simulink model "consolidated_sensors_deploy"  (R2025b)
settings: Solver=FixedStepAuto  StartTime=0.0  StopTime=10.0  RelTol=1e-3  EnableMultiTasking=on
settings Model: ExtModeTrigDuration=2  Creator=atcushen  LastModifiedBy=atcushen
settings SolverCC: PositivePriorityOrder=on
settings OptimizationCC: EnhancedBackFolding=on  PassReuseOutputArgsAs=Individual arguments  ZeroExternalMemoryAtStartup=off  ZeroInternalMemoryAtStartup=off  MaxStackSize=200000  OptimizeBlockOrder=speed  DifferentSizesBufferReuse=on  OptimizationCustomize=off  EfficientTunableParamExpr=on
settings DebuggingCC: ParameterTunabilityLossMsg=error
settings HardwareCC: ProdBitPerPointer=32.0  ProdBitPerSizeT=32.0  ProdBitPerPtrDiffT=32.0  ProdLargestAtomicInteger=Long  ProdLargestAtomicFloat=Double  ProdWordSize=32.0  ProdLongLongMode=on  ProdHWDeviceType=ARM Compatible->ARM Cortex-A (32-bit)  UseEmbeddedCoderFeatures=off  UseSimulinkCoderFeatures=off
settings RTWCC: SystemTargetFile=ert.tlc  HardwareBoard=Raspberry Pi  TLCOptions="-aInlineSetEventsForThisBaseRateFcn=TLC_FALSE -aSuppressMultiTaskScheduler=TLC_FALSE  -aRateBasedStepFcn=0"  TemplateMakefile=ert_default_tmf  Toolchain=GNU GCC Embedded Linux  BuildConfiguration=Faster Runs  Description=Embedded Coder
settings CodeAppCC: ForceParamTrailComments=on  IgnoreCustomStorageClasses=off  OperatorAnnotations=on  SimulinkDataObjDesc=on  SFDataObjDesc=on  InsertBlockDesc=on
settings ERTTargetCC: ExtModeTransport=2.0  ExtModeStaticAlloc=on  ExtModeMexFile=ext_xcp  ExtModeIntrfLevel=Level2 - Open  InlinedParameterPlacement=Hierarchical  SupportNonInlinedSFcns=on  SupportVariableSizeSignals=on

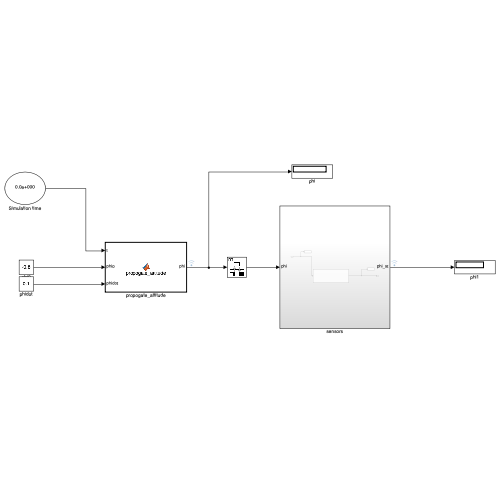
[thumbnail: Simulink's stored preview of the top-level diagram]
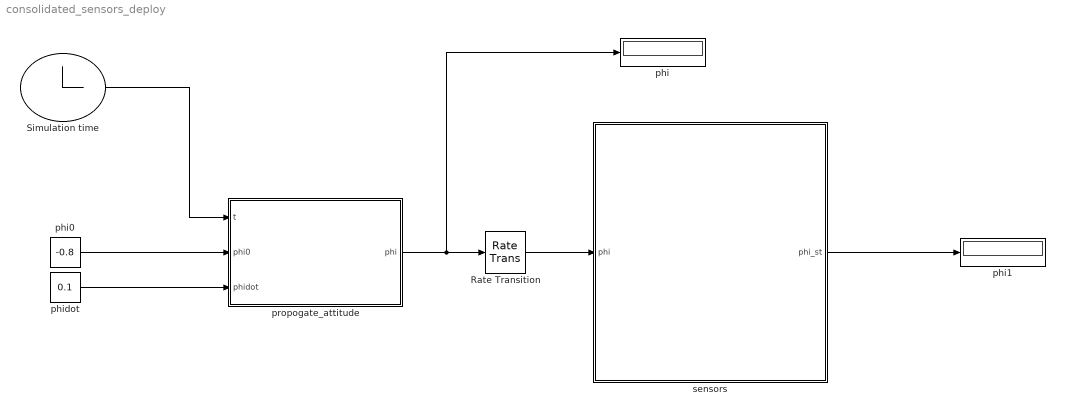
== system consolidated_sensors_deploy ==
  Rate Transition : RateTransition  OutPortSampleTime=0.1
  Simulation time : Clock
  phi : Display
  phi0 : Constant  Value=-0.8
  phi1 : Display
  phidot : Constant  Value=0.1
  propogate_attitude : MATLAB Function  TreatAsAtomicUnit=on
  sensors : Subsystem
  wires:
  Simulation time/1 -> propogate_attitude/1(t)
  propogate_attitude/1(phi) -> phi/1, Rate Transition/1
  phi0/1 -> propogate_attitude/2(phi0)
  phidot/1 -> propogate_attitude/3(phidot)
  Rate Transition/1 -> sensors/1(phi)
  sensors/1(phi_st) -> phi1/1

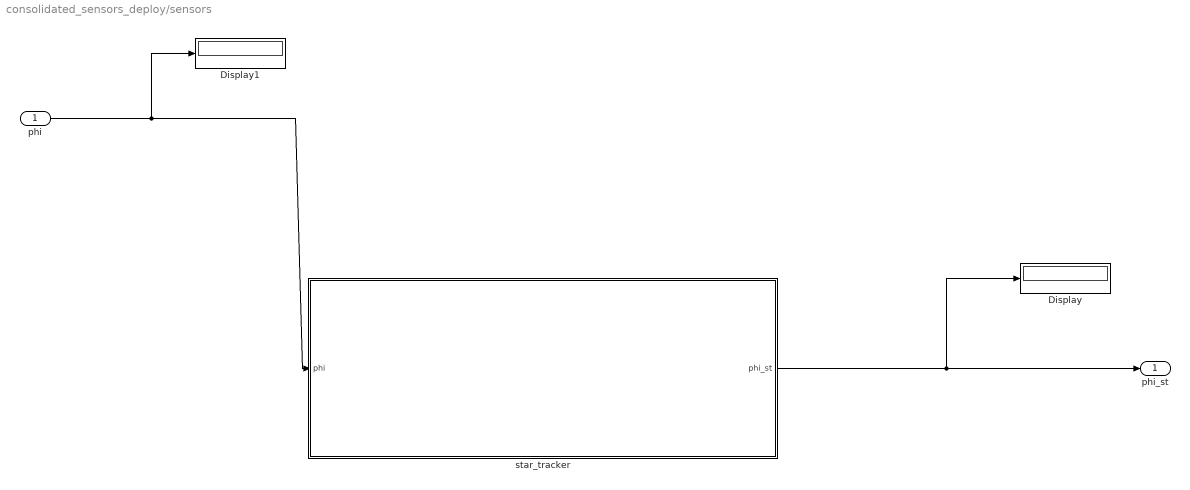
== system consolidated_sensors_deploy/sensors ==
  phi : Inport
  Display : Display
  Display1 : Display
  star_tracker : Subsystem
  phi_st : Outport
  wires:
  phi/1 -> Display1/1, star_tracker/1(phi)
  star_tracker/1(phi_st) -> Display/1, phi_st/1

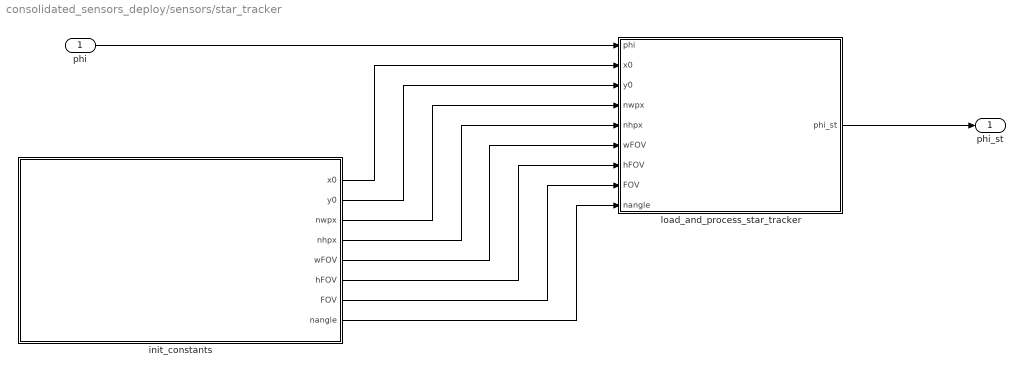
== system consolidated_sensors_deploy/sensors/star_tracker ==
  phi : Inport
  init_constants : MATLAB Function  TreatAsAtomicUnit=on
  load_and_process_star_tracker : MATLAB Function  TreatAsAtomicUnit=on
  phi_st : Outport
  wires:
  load_and_process_star_tracker/1(phi_st) -> phi_st/1
  init_constants/1(x0) -> load_and_process_star_tracker/2(x0)
  phi/1 -> load_and_process_star_tracker/1(phi)
  init_constants/2(y0) -> load_and_process_star_tracker/3(y0)
  init_constants/3(nwpx) -> load_and_process_star_tracker/4(nwpx)
  init_constants/4(nhpx) -> load_and_process_star_tracker/5(nhpx)
  init_constants/5(wFOV) -> load_and_process_star_tracker/6(wFOV)
  init_constants/6(hFOV) -> load_and_process_star_tracker/7(hFOV)
  init_constants/7(FOV) -> load_and_process_star_tracker/8(FOV)
  init_constants/8(nangle) -> load_and_process_star_tracker/9(nangle)

== matlab function consolidated_sensors_deploy/propogate_attitude ==
  data: t input; phi output; phi0 input; phidot input
% propogate attitude
function phi = propogate_attitude(t,phi0,phidot)
    % Input: 
    % t: float, current time, in s
    % phi0: float, initial attitude, in radians
    % phidot: float, rotation rate, in rad/sec
    
    % Output:
    % phi: float, current attitude, in rad/sec

    phi = mod(t*phidot + phi0 + pi,2*pi) - pi;
    %disp(['Propogated attitude at t = ',num2str(t),' to phi = ',num2str(phi)]);
end

== matlab function consolidated_sensors_deploy/sensors/star_tracker/load_and_process_star_tracker ==
  data: phi_st output; phi input; x0 input; y0 input; nwpx input; nhpx input; wFOV input; hFOV input; FOV input; nangle input
function phi_st  = load_and_process_star_tracker(phi,x0,y0,nwpx,nhpx,wFOV,hFOV,FOV,nangle)
    
    % DEFINE PATHS TO STARFIELD IMAGE AND STARTABLE
    starfield_path = 'star_field.mat'; % str, name of reference photo of full starfield image (which nwpx,wFOV etc describe)
    startable_path = 'star_table.mat'; % str, name of table which identifies star locations, in radians 


    % PART 1: IMPORT STAR TABLE

    struct = coder.load(startable_path);
    star_table = struct.star_table;
    

    
    % PART 2: GENERATE LOOKUP TABLE

    % Initialize lookup table
    star_lookup = zeros(size(star_table, 1), nangle);

    % Iterate through each star in the table
    for istar = 1:length(star_table)
        
        % Compute the angular distances from the current star to all other stars
        phi_diff = star_table(istar, 1) - star_table(:, 1);
        theta_diff = star_table(istar, 2) - star_table(:, 2);
        angle_diff = sqrt(phi_diff.^2 + theta_diff.^2);

        % Sort the angular distances and get the indices of the smallest values
        [sorted_angles, ~] = sort(angle_diff);
        star_lookup(istar, :) = sorted_angles(2:min(nangle+1, length(sorted_angles))); % Store the smallest values
    end

    
    % PART 3: LOAD AND CROP IMAGE

    % Input
    % image: str, path to .png field to import of starfield
    % phi: float, boresight angle of camera, in radians, from -pi to pis
    % FOV: float, angular field of view of camera, in radians, from 0 to 2pi
    % x0: int, x pixel coord of reference star 
    % y0: int, x pixel coord of reference star 
    % nwpx: int, number of pixels of width of starfield image
    % nhpx: int, number of pixels of height of starfield image
    % wFOV: float, field of view width of starfield image [deg]
    % hFOV: float, field of view height of starfield image [deg]
    % Output:
    % st_im: nres x nres array, representing synethic star tracker image

    % Load the .png image as a black and white image array
    file = coder.load(starfield_path);
    img = file.img; 
    starfield_im = rgb2gray(img); % Convert the image to grayscale
    starfield_im = flip(starfield_im,1); % Image array is upside down)

    % Create coordinate axes
    x_ax = linspace(1,nwpx,nwpx) - x0;
    y_ax = linspace(1,nhpx,nhpx) - y0;
    phi_ax = x_ax * pi/180 * wFOV/nwpx;
    theta_ax = y_ax * pi/180 * hFOV/nhpx;
    
    % Crop the starfield image based on the field of view and the phi axis
    phi_indices = phi_ax >= (phi - FOV/2) & phi_ax <= (phi + FOV/2);
    theta_indices = theta_ax >= (-FOV/2) & theta_ax <= (FOV/2); %y0-round(nres/2):y0-round(nres/2)+nres-1;
    
    % Ensure indices are within bounds
    %phi_indices = max(min(phi_indices, nwpx), 1);
    %theta_indices = max(min(theta_indices, nhpx), 1);
    
    % Crop the image
    st_im = starfield_im(theta_indices, phi_indices);

    
    % PART 4: LOCATE STARS

    % Input:
    % st_im: nxn array, representing image from star tracker
    % FOV: float, field of view along each edge of image
    % Output:
    % star_ls: nx2 array, the phi and theta positions (relative to the
    % center of the image) for each star identified
    
    % Get image dimensions (not passed to function call)
    [theta_nres,phi_nres] = size(st_im);
    
    % Convert coordinates to phi and theta positions
    phi_positions = linspace(-FOV/2, FOV/2, phi_nres);
    theta_positions = linspace(-FOV/2, FOV/2, theta_nres);
    
    % Identify bright points in the star tracker image
     threshold = 0.3 * 255; % Set a threshold to identify bright points
    % Create filtered im
     filtered_im = zeros(size(st_im)); % Initialize filtered image
     filtered_im(st_im > threshold) = 1; % Set values to 1 where st_im exceeds threshold
    % Find connected components
     CC = bwconncomp(filtered_im);
    % Create label matrix - CHANGED FOR CODEGEN
     L = zeros(size(filtered_im), 'uint16');
     for k = 1:CC.NumObjects
         L(CC.PixelIdxList{k}) = k;
     end
    % Create output array for star positions
     star_ls = zeros(max(L(:)), 2);
    % Iterate through each connected component
    for istar = 1:max(L(:))
    % Get the coordinates of the current star cluster
     [y_cluster, x_cluster] = find(L == istar);
    % Store the average position of the cluster
     star_ls(istar, 1) = mean(phi_positions(x_cluster)); % Average phi coordinate
     star_ls(istar, 2) = mean(theta_positions(y_cluster)); % Average theta coordinate
    end
    

    % PART 5: MATCH STARS TO LOOKUP TABLE

    star_pos_error = 10*wFOV/nwpx*pi/180;

    % Input
    % star_ls: nx2 array, the phi and theta positions (relative to the
    % center of the image) for each star identified
    % star_pos_error: float, angular uncertainty in position of stars
    % star_lookup: nxnagle array, each row corresponds to given row in
    % star_table, columns are angular distances to closest stars

    % Output
    % star_num: integer, index number of matched star
    % deltaphi: float, offset in phi of matched star from image center, in
    % radians
    % deltatheta: float, offset in phi of matched star from image center,
    % in radians
    % CHANGED FOR CODEGEN - Initialize outputs with default values
    star_num = int32(-1);
    deltaphi = 0.0;
    deltatheta = 0.0;
    match_status = int32(0);  % debug output
    stars_tried = int32(0);   % debug output

    % Iterate through stars in image, starting closest to middle, until we
    % get a positive match
    star_match = false;
    
    % Calculate the sum of squares for each star position
    star_ls_dist = sum(star_ls.^2, 2);
    
    % Sort the star_ls based on the sum of squares
    [~, sorted_indices] = sort(star_ls_dist);
    star_ls = star_ls(sorted_indices, :);

    istar = 1;
    while star_match == false && istar <= length(star_ls)
        stars_tried = int32(istar);  % tracking progress
        
        % Compute distances to other stars
        phi_diff = star_ls(istar, 1) - star_ls(:, 1);
        theta_diff = star_ls(istar, 2) - star_ls(:, 2);
        angle_diff = sqrt(phi_diff.^2 + theta_diff.^2);

        % Sort the computed angular distances from smallest to largest
        [sorted_angles, ~] = sort(angle_diff);
        
        % Drop the first element of sorted_angles (distance to itself = 0)
        sorted_angles(1) = [];

        % Reduce sorted angles to only be as long as star_lookup is wide
        sorted_angles = sorted_angles(1:min(length(sorted_angles), size(star_lookup, 2)));

        % Create an array of stars within the positional error range
        match_indices = star_lookup(:, 1) >= (sorted_angles(1) - star_pos_error) & ...
                        star_lookup(:, 1) <= (sorted_angles(1) + star_pos_error);
        matched_stars = star_lookup(match_indices, :);

        % Check if that immediately identified the current state. 
        % If not, compare the angular distances one by one, bringing in more to
        % reduce the number of remaining options
        iangle = 2;

        while size(matched_stars,1) > 1 & iangle <= size(star_lookup,2)
            match_status = int32(2);  % indicates multiple matches being refined
            
            % We loop through the remaining matches
            for j = 1:size(match_indices, 1)
                if j ~= 0
                    % Check to see if the next closest star is within error of
                    % any of the neighbouring stars listed in the lookup table
                    % If none of the angles are close enough, then reject this
                    % match
                    if all(abs(star_lookup(j, iangle:end) - sorted_angles(iangle)) > star_pos_error)
                        match_indices(j) = 0; % Set the jth non-zero element of match_indices to zero
                    end
                end 
            end
            matched_stars = star_lookup(match_indices, :);
        
            iangle = iangle + 1;
        end
        
        % Check if we could use this star 
        if size(matched_stars,1) ~= 1
            % no match found for this star, continue
            istar = istar + 1; % Move to the next star
        else
            % CHANGED FOR CODEGEN - Force scalar by using loop instead of find
            for k = 1:length(match_indices)
                if match_indices(k) ~= 0
                    star_num = int32(k)
                    break;
                end
            end
            deltaphi = star_ls(istar,1); % Offset in phi
            deltatheta = star_ls(istar,2); % Offset in theta
            star_match = true;
            match_status = int32(1);  % successful match
        end
    end
    
    % Return error if star tracker failed 
    if star_match == false
        % CHANGED FOR CODEGEN - tracker failed
        star_num = int32(-1);
        deltaphi = 0.0;
        deltatheta = 0.0;
        match_status = int32(0);  % Failed to match
    end


    % FINALLY, COMPUTE PHI_ST

    if star_num<0
        phi_st = NaN;
    else
        phi_st = star_table(star_num,1) - deltaphi;
    end

end

== matlab function consolidated_sensors_deploy/sensors/star_tracker/init_constants ==
  data: x0 output; y0 output; nwpx output; nhpx output; wFOV output; hFOV output; FOV output; nangle output
% define all our constants
function [x0,y0,nwpx,nhpx,wFOV,hFOV,FOV,nangle] = init_constants
    % Output
    x0 = 3270;  % int, pixel coords of reference star used to set phi=0
    y0 = 1608; % int, pixel coords of reference star used to set theta=0
    nwpx = 4608; % int, pixel width of full starfield image
    nhpx = 2592; % int, pixel height of full starfield image
    wFOV = 102; % float, angular field of view of reference starfield image width, in degrees
    hFOV = 67; % float, angular field of view of reference starfield image height, in degrees
    FOV = pi/6; % float, chosen field of fiew of cropped starfield image, in radians
    nangle = 12; % int, how many angular distances to compute for each star
end
